simulink model "Problem_5"  (R2020b)
settings: Solver=VariableStepAuto  StartTime=0.0  StopTime=10.0  RelTol=1e-3
settings Model: Creator=sonal  LastModifiedBy=sonal

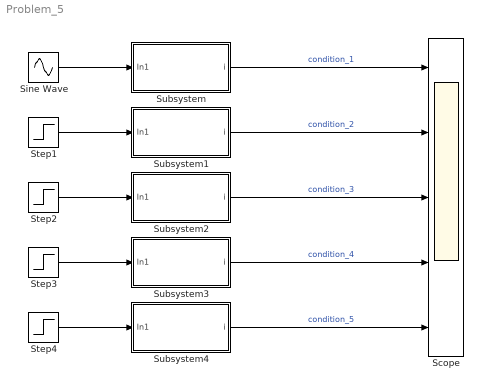
== system Problem_5 ==
  Scope : Scope  NumInputPorts=5
  Sine Wave : Sin  SampleTime=0
  Step1 : Step  Before=2  After=5  SampleTime=0
  Step2 : Step  Time=2  Before=3  After=13  SampleTime=0
  Step3 : Step  Before=4  After=14  SampleTime=0
  Step4 : Step  Before=5  After=15  SampleTime=0
  Subsystem : Subsystem
  Subsystem1 : Subsystem
  Subsystem2 : Subsystem
  Subsystem3 : Subsystem
  Subsystem4 : Subsystem
  wires:
  Sine Wave/1 -> Subsystem/1(In1)
  Step1/1 -> Subsystem1/1(In1)
  Step4/1 -> Subsystem4/1(In1)
  Subsystem1/1(i) -> Scope/2  "condition_2"
  Subsystem3/1(i) -> Scope/4  "condition_4"
  Subsystem4/1(i) -> Scope/5  "condition_5"
  Step2/1 -> Subsystem2/1(In1)
  Subsystem/1(i) -> Scope/1  "condition_1"
  Subsystem2/1(i) -> Scope/3  "condition_3"
  Step3/1 -> Subsystem3/1(In1)

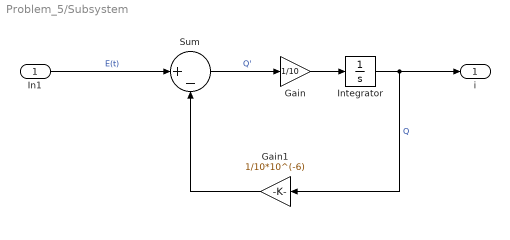
== system Problem_5/Subsystem ==
  In1 : Inport
  Gain : Gain  Gain=1/10
  Gain1 : Gain  Gain=1/10*10^(-6)
  Integrator : Integrator
  Sum : Sum  Inputs=|+-
  i : Outport
  wires:
  In1/1 -> Sum/1  "E(t)"
  Sum/1 -> Gain/1  "Q'"
  Gain1/1 -> Sum/2
  Integrator/1 -> i/1, Gain1/1  "Q"
  Gain/1 -> Integrator/1

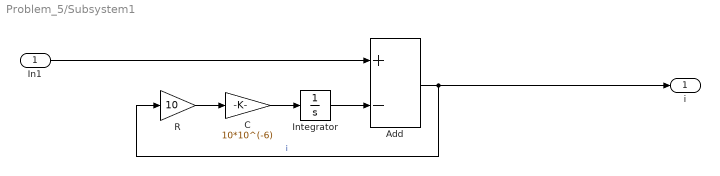
== system Problem_5/Subsystem1 ==
  In1 : Inport
  Add : Sum  Inputs=+-
  C : Gain  Gain=10*10^(-6)
  Integrator : Integrator
  R : Gain  Gain=10
  i : Outport
  wires:
  Add/1 -> R/1, i/1  "i"
  In1/1 -> Add/1
  Integrator/1 -> Add/2
  C/1 -> Integrator/1
  R/1 -> C/1

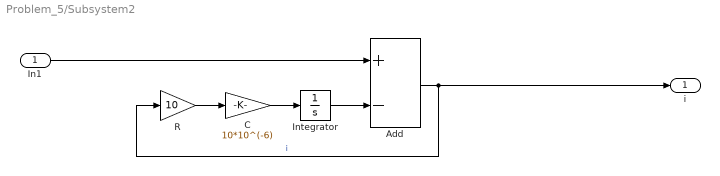
== system Problem_5/Subsystem2 ==
  In1 : Inport
  Add : Sum  Inputs=+-
  C : Gain  Gain=10*10^(-6)
  Integrator : Integrator
  R : Gain  Gain=10
  i : Outport
  wires:
  R/1 -> C/1
  C/1 -> Integrator/1
  Integrator/1 -> Add/2
  In1/1 -> Add/1
  Add/1 -> i/1, R/1  "i"

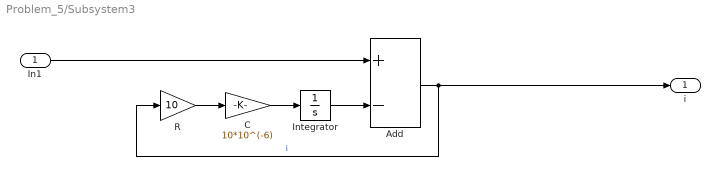
== system Problem_5/Subsystem3 ==
  In1 : Inport
  Add : Sum  Inputs=+-
  C : Gain  Gain=10*10^(-6)
  Integrator : Integrator
  R : Gain  Gain=10
  i : Outport
  wires:
  Add/1 -> R/1, i/1  "i"
  In1/1 -> Add/1
  Integrator/1 -> Add/2
  C/1 -> Integrator/1
  R/1 -> C/1

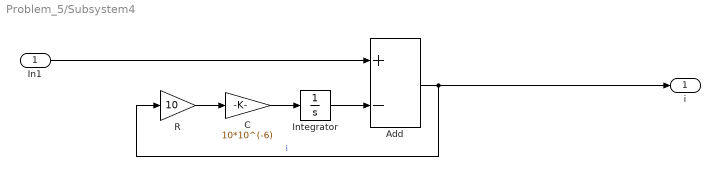
== system Problem_5/Subsystem4 ==
  In1 : Inport
  Add : Sum  Inputs=+-
  C : Gain  Gain=10*10^(-6)
  Integrator : Integrator
  R : Gain  Gain=10
  i : Outport
  wires:
  R/1 -> C/1
  C/1 -> Integrator/1
  Integrator/1 -> Add/2
  In1/1 -> Add/1
  Add/1 -> i/1, R/1  "i"
